simulink model "robatic_lander"  (R2023b)
settings: Solver=VariableStepAuto  StartTime=0.0  StopTime=10  MaxStep=1/400  RelTol=1e-3
values from neighbouring files (symbols this model uses):
  A = 5.03e-6    (= 5.03e-06)    [params.m]
  Ae = pi * (3.62e-6^2) / 4    (= 1.02921716924e-11)    [params.m]
  g_sea = 9.80665    [params.m]
  gam = 1.4    [params.m]
  lapse_rate = 6.5    [params.m]
  lever_arm = 1    [params.m]
  m = (m_tube_avg + m_frame)    (= 36)    [params.m]
  Me = 2.2    [params.m]
  molar_mass_air = 0.0289644    [params.m]
  P0 = 101325    [params.m]
  R = 287.05    [params.m]
  R_const = 8.31432    [params.m]
  re = 6371009    [params.m]
  sea_level_temp_c = 15    [params.m]
  sea_level_temp_k = sea_level_temp_c + 274.15    (= 289.15)    [params.m]
libraries: shared6dof x1, simulink_extras x1
settings Model: Creator=yigit  LastModifiedBy=yigit

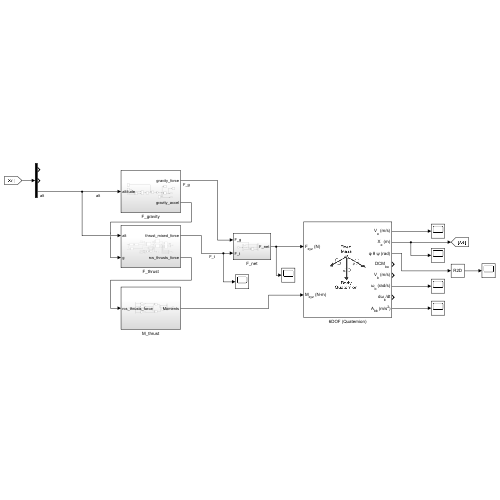
[thumbnail: Simulink's stored preview of the top-level diagram]
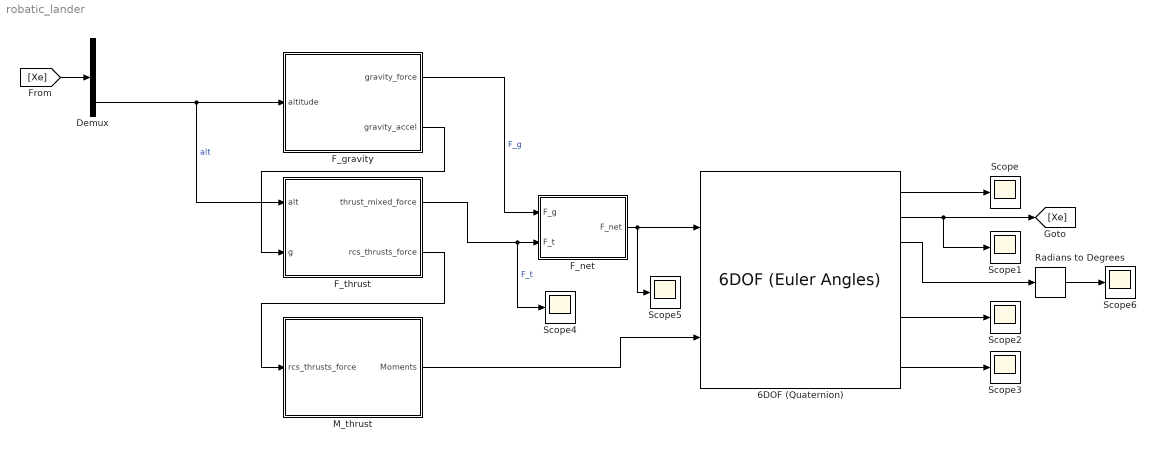
== system robatic_lander ==
  6DOF (Quaternion) : shared6dof/6DOF (Euler Angles)  units=Metric (MKS)  mtype=Fixed  rep=Quaternion  xme_0=init_pos  Vm_0=init_vel_body  eul_0=init_eulr  pm_0=init_pqr  mass_0=m  mass_e=0.5  mass_f=2.0  inertia=I  inertia_e=eye(3)  inertia_f=2*eye(3)  k_quat=1.0  vre_flag=on  abi_flag=off  aMode=0  xme_statename=''  Vm_statename=''  eul_statename=''  quat_statename=''  pm_statename=''  mass_statename=''
      settings: LibrarySourceBlock=aerolib6dof2/6DOF (Quaternion)
  Demux : Demux  Outputs=3
  F_gravity : Subsystem
  F_net : Subsystem
  F_thrust : Subsystem
  M_thrust : Subsystem
  Radians to Degrees : simulink_extras/Transformations/Radians to Degrees
  Scope{,1..6} (7 alike) : Scope
  wires:
  F_thrust/2(rcs_thrusts_force) -> M_thrust/1(rcs_thrusts_force)
  M_thrust/1(Moments) -> 6DOF (Quaternion)/2
  6DOF (Quaternion)/1 -> Scope/1
  6DOF (Quaternion)/2 -> [Xe], Scope1/1
  6DOF (Quaternion)/6 -> Scope2/1
  6DOF (Quaternion)/8 -> Scope3/1
  [Xe] -> Demux/1
  Demux/3 -> F_thrust/1(alt), F_gravity/1(altitude)  "alt"
  F_thrust/1(thrust_mixed_force) -> Scope4/1, F_net/2(F_t)  "F_t"
  F_net/1(F_net) -> Scope5/1, 6DOF (Quaternion)/1
  F_gravity/1(gravity_force) -> F_net/1(F_g)  "F_g"
  F_gravity/2(gravity_accel) -> F_thrust/2(g)
  6DOF (Quaternion)/3 -> Radians to Degrees/1
  Radians to Degrees/1 -> Scope6/1

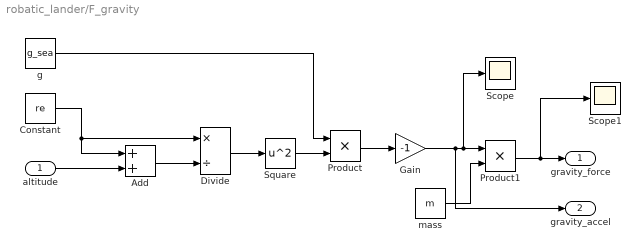
== system robatic_lander/F_gravity ==
  altitude : Inport
  Add : Sum
  Constant : Constant  Value=re
  Divide : Product  Inputs=*/
  Gain : Gain  Gain=-1
  Product : Product
  Product1 : Product
  Scope : Scope
  Scope1 : Scope
  Square : Math  Operator=square
  g : Constant  Value=g_sea
  mass : Constant  Value=m
  gravity_force : Outport
  gravity_accel : Outport  Port=2
  wires:
  Constant/1 -> Add/1, Divide/1
  Add/1 -> Divide/2
  altitude/1 -> Add/2
  Square/1 -> Product/2
  g/1 -> Product/1
  Product/1 -> Gain/1
  mass/1 -> Product1/2
  Product1/1 -> Scope1/1, gravity_force/1
  Divide/1 -> Square/1
  Gain/1 -> gravity_accel/1, Scope/1, Product1/1

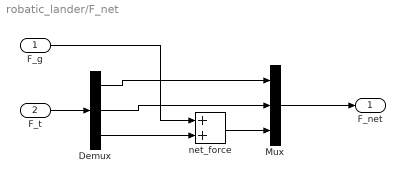
== system robatic_lander/F_net ==
  F_g : Inport
  F_t : Inport  Port=2
  Demux : Demux  Outputs=3
  Mux : Mux  Inputs=3
  net_force : Sum
  F_net : Outport
  wires:
  F_t/1 -> Demux/1
  Demux/3 -> net_force/2
  F_g/1 -> net_force/1
  Mux/1 -> F_net/1
  Demux/1 -> Mux/1
  net_force/1 -> Mux/3
  Demux/2 -> Mux/2

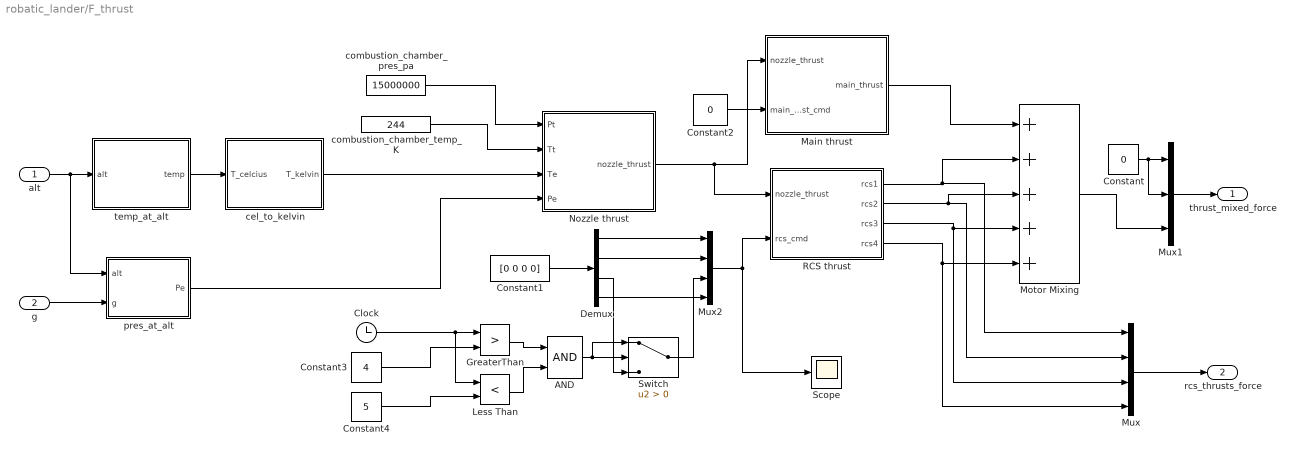
== system robatic_lander/F_thrust ==
  alt : Inport
  g : Inport  Port=2
  AND : Logic  IconShape=distinctive  AllPortsSameDT=off  OutDataTypeStr=boolean
  Clock : Clock
  Constant : Constant  Value=0
  Constant1 : Constant  Value=[0 0 0 0]
  Constant2 : Constant  Value=0
  Constant3 : Constant  Value=4
  Constant4 : Constant  Value=5
  Demux : Demux
  GreaterThan : RelationalOperator  Operator=>  OutDataTypeStr=boolean  RndMeth=Simplest  InputSameDT=off
  Less Than : RelationalOperator  Operator=<  OutDataTypeStr=boolean  RndMeth=Simplest  InputSameDT=off
  Main thrust : Subsystem
  Motor Mixing : Sum  Inputs=+++++
  Mux : Mux
  Mux1 : Mux  Inputs=3
  Mux2 : Mux
  Nozzle thrust : Subsystem
  RCS thrust : Subsystem
  Scope : Scope
  Switch : Switch  Criteria=u2 > Threshold  SaturateOnIntegerOverflow=off  InputSameDT=off
  cel_to_kelvin : Subsystem
  combustion_chamber_pres_pa : Constant  Value=15000000
  combustion_chamber_temp_K : Constant  Value=244
  pres_at_alt : Subsystem
  temp_at_alt : Subsystem
  thrust_mixed_force : Outport
  rcs_thrusts_force : Outport  Port=2
  wires:
  Main thrust/1(main_thrust) -> Motor Mixing/1
  RCS thrust/1(rcs1) -> Mux/1, Motor Mixing/2
  RCS thrust/2(rcs2) -> Mux/2, Motor Mixing/3
  RCS thrust/3(rcs3) -> Mux/3, Motor Mixing/4
  RCS thrust/4(rcs4) -> Mux/4, Motor Mixing/5
  Mux/1 -> rcs_thrusts_force/1
  Mux1/1 -> thrust_mixed_force/1
  Motor Mixing/1 -> Mux1/3
  Constant/1 -> Mux1/2, Mux1/1
  Nozzle thrust/1(nozzle_thrust) -> Main thrust/1(nozzle_thrust), RCS thrust/1(nozzle_thrust)
  combustion_chamber_pres_pa/1 -> Nozzle thrust/1(Pt)
  combustion_chamber_temp_K/1 -> Nozzle thrust/2(Tt)
  alt/1 -> pres_at_alt/1(alt), temp_at_alt/1(alt)
  g/1 -> pres_at_alt/2(g)
  pres_at_alt/1(Pe) -> Nozzle thrust/4(Pe)
  temp_at_alt/1(temp) -> cel_to_kelvin/1(T_celcius)
  cel_to_kelvin/1(T_kelvin) -> Nozzle thrust/3(Te)
  Constant2/1 -> Main thrust/2(main_thrust_cmd)
  Constant1/1 -> Demux/1
  Mux2/1 -> RCS thrust/2(rcs_cmd), Scope/1
  Demux/1 -> Mux2/1
  Demux/2 -> Mux2/2
  Demux/4 -> Mux2/4
  Clock/1 -> Less Than/1, GreaterThan/1
  Constant3/1 -> GreaterThan/2
  Constant4/1 -> Less Than/2
  GreaterThan/1 -> AND/1
  Less Than/1 -> AND/2
  AND/1 -> Switch/1, Switch/2
  Demux/3 -> Switch/3
  Switch/1 -> Mux2/3

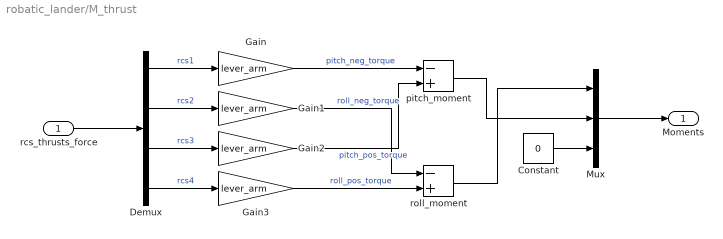
== system robatic_lander/M_thrust ==
  rcs_thrusts_force : Inport
  Constant : Constant  Value=0
  Demux : Demux
  Gain{,1..3} (4 alike) : Gain  Gain=lever_arm
  Mux : Mux  Inputs=3
  pitch_moment : Sum  Inputs=-+
  roll_moment : Sum  Inputs=-+
  Moments : Outport
  wires:
  rcs_thrusts_force/1 -> Demux/1
  Demux/1 -> Gain/1  "rcs1"
  Demux/2 -> Gain1/1  "rcs2"
  Demux/3 -> Gain2/1  "rcs3"
  Demux/4 -> Gain3/1  "rcs4"
  Gain1/1 -> roll_moment/1  "roll_neg_torque"
  Gain3/1 -> roll_moment/2  "roll_pos_torque"
  Gain/1 -> pitch_moment/1  "pitch_neg_torque"
  Gain2/1 -> pitch_moment/2  "pitch_pos_torque"
  Mux/1 -> Moments/1
  roll_moment/1 -> Mux/1
  pitch_moment/1 -> Mux/2
  Constant/1 -> Mux/3

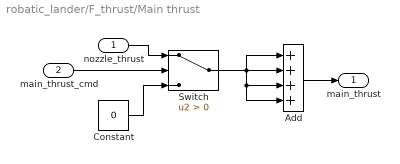
== system robatic_lander/F_thrust/Main thrust ==
  nozzle_thrust : Inport
  main_thrust_cmd : Inport  Port=2
  Add : Sum  Inputs=++++
  Constant : Constant  Value=0
  Switch : Switch  Criteria=u2 > Threshold  SaturateOnIntegerOverflow=off  InputSameDT=off
  main_thrust : Outport
  wires:
  Add/1 -> main_thrust/1
  Switch/1 -> Add/4, Add/3, Add/1, Add/2
  main_thrust_cmd/1 -> Switch/2
  nozzle_thrust/1 -> Switch/1
  Constant/1 -> Switch/3

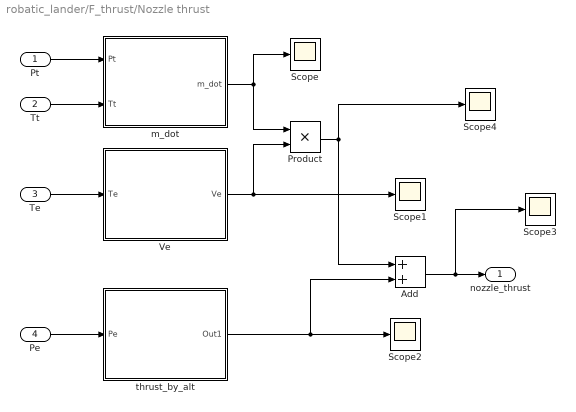
== system robatic_lander/F_thrust/Nozzle thrust ==
  Pt : Inport
  Tt : Inport  Port=2
  Te : Inport  Port=3
  Pe : Inport  Port=4
  Add : Sum
  Product : Product
  Scope{,1..4} (5 alike) : Scope
  Ve : Subsystem
  m_dot : Subsystem
  thrust_by_alt : Subsystem
  nozzle_thrust : Outport
  wires:
  Pt/1 -> m_dot/1(Pt)
  Tt/1 -> m_dot/2(Tt)
  m_dot/1(m_dot) -> Scope/1, Product/1
  Product/1 -> Scope4/1, Add/1
  Add/1 -> Scope3/1, nozzle_thrust/1
  Ve/1(Ve) -> Scope1/1, Product/2
  Te/1 -> Ve/1(Te)
  thrust_by_alt/1(Out1) -> Scope2/1, Add/2
  Pe/1 -> thrust_by_alt/1(Pe)

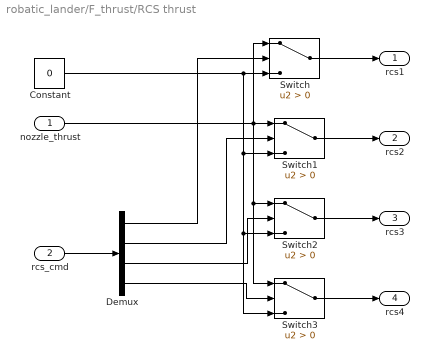
== system robatic_lander/F_thrust/RCS thrust ==
  nozzle_thrust : Inport
  rcs_cmd : Inport  Port=2
  Constant : Constant  Value=0
  Demux : Demux
  Switch{,1..3} (4 alike) : Switch  Criteria=u2 > Threshold  SaturateOnIntegerOverflow=off  InputSameDT=off
  rcs1 : Outport
  rcs2 : Outport  Port=2
  rcs3 : Outport  Port=3
  rcs4 : Outport  Port=4
  wires:
  Switch/1 -> rcs1/1
  Switch1/1 -> rcs2/1
  Switch2/1 -> rcs3/1
  Switch3/1 -> rcs4/1
  Demux/1 -> Switch/2
  Demux/2 -> Switch1/2
  Demux/3 -> Switch2/2
  Demux/4 -> Switch3/2
  rcs_cmd/1 -> Demux/1
  nozzle_thrust/1 -> Switch/1, Switch1/1, Switch3/1, Switch2/1
  Constant/1 -> Switch1/3, Switch3/3, Switch2/3, Switch/3

== system robatic_lander/F_thrust/cel_to_kelvin ==
  T_celcius : Inport
  Add : Sum
  Constant : Constant  Value=273.15
  T_kelvin : Outport
  wires:
  T_celcius/1 -> Add/1
  Add/1 -> T_kelvin/1
  Constant/1 -> Add/2

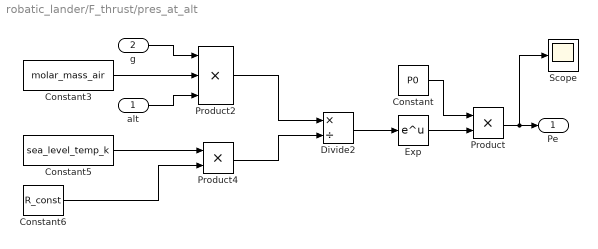
== system robatic_lander/F_thrust/pres_at_alt ==
  alt : Inport
  g : Inport  Port=2
  Constant : Constant  Value=P0
  Constant3 : Constant  Value=molar_mass_air
  Constant5 : Constant  Value=sea_level_temp_k
  Constant6 : Constant  Value=R_const
  Divide2 : Product  Inputs=*/
  Exp : Math
  Product : Product
  Product2 : Product  Inputs=3
  Product4 : Product
  Scope : Scope
  Pe : Outport
  wires:
  Product/1 -> Scope/1, Pe/1
  Constant/1 -> Product/1
  g/1 -> Product2/1
  Constant3/1 -> Product2/2
  Exp/1 -> Product/2
  Divide2/1 -> Exp/1
  Product2/1 -> Divide2/1
  alt/1 -> Product2/3
  Product4/1 -> Divide2/2
  Constant5/1 -> Product4/1
  Constant6/1 -> Product4/2

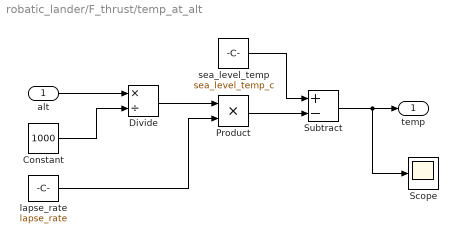
== system robatic_lander/F_thrust/temp_at_alt ==
  alt : Inport
  Constant : Constant  Value=1000
  Divide : Product  Inputs=*/
  Product : Product
  Scope : Scope
  Subtract : Sum  Inputs=+-
  lapse_rate : Constant  Value=lapse_rate
  sea_level_temp : Constant  Value=sea_level_temp_c
  temp : Outport
  wires:
  alt/1 -> Divide/1
  Constant/1 -> Divide/2
  Divide/1 -> Product/1
  lapse_rate/1 -> Product/2
  Product/1 -> Subtract/2
  sea_level_temp/1 -> Subtract/1
  Subtract/1 -> Scope/1, temp/1

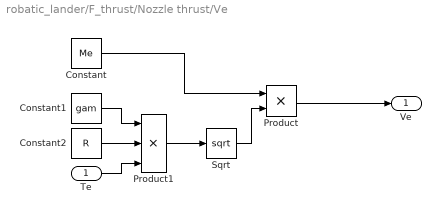
== system robatic_lander/F_thrust/Nozzle thrust/Ve ==
  Te : Inport
  Constant : Constant  Value=Me
  Constant1 : Constant  Value=gam
  Constant2 : Constant  Value=R
  Product : Product
  Product1 : Product  Inputs=3
  Sqrt : Sqrt
  Ve : Outport
  wires:
  Constant/1 -> Product/1
  Product/1 -> Ve/1
  Product1/1 -> Sqrt/1
  Sqrt/1 -> Product/2
  Te/1 -> Product1/3
  Constant2/1 -> Product1/2
  Constant1/1 -> Product1/1

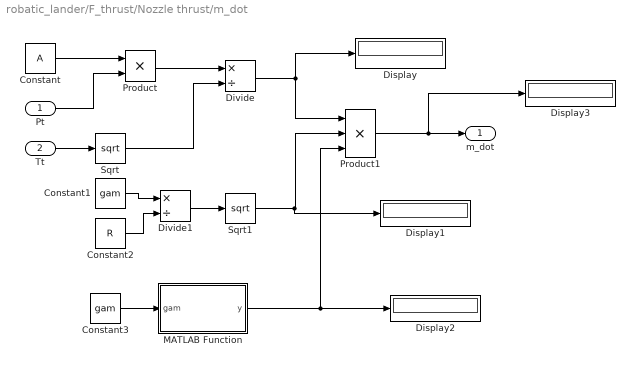
== system robatic_lander/F_thrust/Nozzle thrust/m_dot ==
  Pt : Inport
  Tt : Inport  Port=2
  Constant : Constant  Value=A
  Constant1 : Constant  Value=gam
  Constant2 : Constant  Value=R
  Constant3 : Constant  Value=gam
  Display{,1..3} (4 alike) : Display
  Divide : Product  Inputs=*/
  Divide1 : Product  Inputs=*/
  MATLAB Function : MATLAB Function  TreatAsAtomicUnit=on
  Product : Product
  Product1 : Product  Inputs=3
  Sqrt : Sqrt
  Sqrt1 : Sqrt
  m_dot : Outport
  wires:
  Constant/1 -> Product/1
  Pt/1 -> Product/2
  Product/1 -> Divide/1
  Tt/1 -> Sqrt/1
  Sqrt/1 -> Divide/2
  Divide1/1 -> Sqrt1/1
  Constant1/1 -> Divide1/1
  Constant2/1 -> Divide1/2
  Divide/1 -> Display/1, Product1/1
  Sqrt1/1 -> Display1/1, Product1/2
  MATLAB Function/1(y) -> Product1/3, Display2/1
  Product1/1 -> Display3/1, m_dot/1
  Constant3/1 -> MATLAB Function/1(gam)

== system robatic_lander/F_thrust/Nozzle thrust/thrust_by_alt ==
  Pe : Inport
  Constant : Constant  Value=P0
  Constant1 : Constant  Value=Ae
  Product : Product
  Subtract : Sum  Inputs=+-
  Out1 : Outport
  wires:
  Pe/1 -> Subtract/1
  Constant/1 -> Subtract/2
  Subtract/1 -> Product/1
  Product/1 -> Out1/1
  Constant1/1 -> Product/2

== matlab function robatic_lander/F_thrust/Nozzle thrust/m_dot/MATLAB Function ==
  data: gam input; y output
function y = fcn(gam)
y = ((gam + 1) / 2) ^ (- ( (gam + 1) / (2 * (gam - 1)) ) );
